simulink model "MotorCntrl"  (R2020b)
settings: Solver=ode45  StartTime=0.0  StopTime=0.4  RelTol=1e-3
undefined symbols (not defined in the file): b, J, Ke, Kt, L, R
settings Model: DataDictionary=Motor_DataDictionary.sldd  Creator=Sourav Kumar  LastModifiedBy=Makrand Raut Dessai

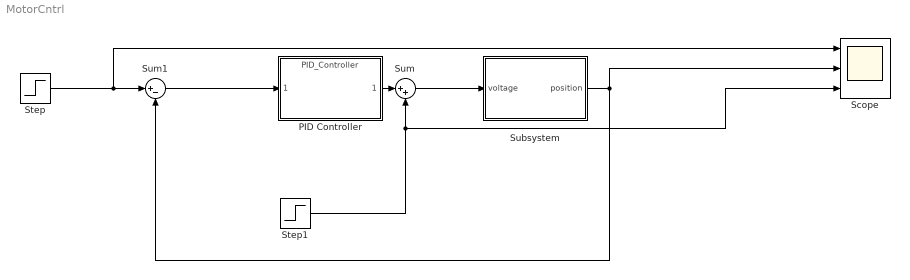
== system MotorCntrl ==
  PID Controller : ModelReference  ModelNameDialog=PID_Controller  SimulationMode=Normal  ModelReferenceVersion=1.4
  Scope : Scope  NumInputPorts=3
  Step : Step  Time=0  SampleTime=0
  Step1 : Step  Time=0.01  SampleTime=0
  Subsystem : Subsystem
  Sum : Sum  Inputs=|++
  Sum1 : Sum  Inputs=|+-
  wires:
  Step/1 -> Scope/1, Sum1/1
  Sum1/1 -> PID Controller/1
  PID Controller/1 -> Sum/1
  Sum/1 -> Subsystem/1(voltage)
  Step1/1 -> Sum/2, Scope/3
  Subsystem/1(position) -> Sum1/2, Scope/2

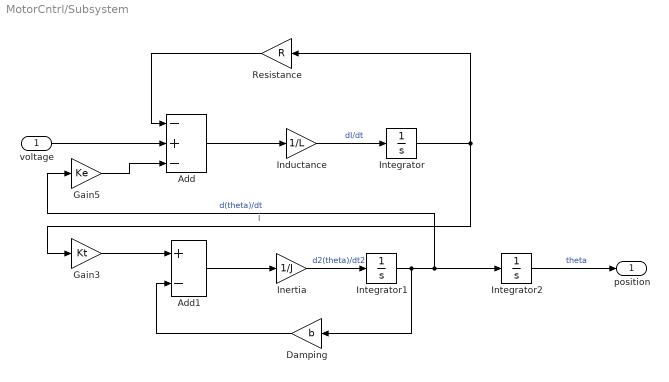
== system MotorCntrl/Subsystem ==
  voltage : Inport
  Add : Sum  Inputs=-+-
  Add1 : Sum  Inputs=+-
  Damping : Gain  Gain=b
  Gain3 : Gain  Gain=Kt
  Gain5 : Gain  Gain=Ke
  Inductance : Gain  Gain=1/L
  Inertia : Gain  Gain=1/J
  Integrator : Integrator
  Integrator1 : Integrator
  Integrator2 : Integrator
  Resistance : Gain  Gain=R
  position : Outport
  wires:
  Integrator1/1 -> Damping/1, Gain5/1, Integrator2/1  "d(theta)/dt"
  Add/1 -> Inductance/1
  Inductance/1 -> Integrator/1  "dI/dt"
  Integrator/1 -> Gain3/1, Resistance/1  "I"
  Resistance/1 -> Add/1
  voltage/1 -> Add/2
  Add1/1 -> Inertia/1
  Integrator2/1 -> position/1  "theta"
  Damping/1 -> Add1/2
  Gain5/1 -> Add/3
  Inertia/1 -> Integrator1/1  "d2(theta)/dt2"
  Gain3/1 -> Add1/1
